simulink model "Bleed_TestBed1"  (R2019b)
settings: Solver=FixedStepDiscrete  StartTime=0.0  StopTime=1  FixedStep=1  RelTol=1e-3  EnableMultiTasking=on
undefined symbols (not defined in the file): MWS
libraries: Lib_Turbo_Bleed_TMATS x1
settings Model: Creator=jwchapm2  LastModifiedBy=bhisma
settings DataIOCC: LimitDataPoints=on  SaveFormat=Array  ReturnWorkspaceOutputs=off
settings OptimizationCC: ExpressionDepthLimit=2147483647  LifeSpan=inf
settings DebuggingCC: UnderspecifiedInitializationDetection=Classic  MergeDetectMultiDrivingBlocksExec=none  SolverPrmCheckMsg=warning  StateNameClashWarn=warning  SFUnexpectedBacktrackingDiag=warning  SFNoUnconditionalDefaultTransitionDiag=warning  SFExecutionAtInitializationDiag=none  ArithmeticOperatorsInVariantConditions=warning
settings HardwareCC: ProdBitPerPointer=32  ProdBitPerSizeT=32  ProdBitPerPtrDiffT=32  ProdLargestAtomicFloat=None  ProdIntDivRoundTo=Undefined  ProdEndianess=Unspecified  ProdWordSize=32  ProdHWDeviceType=32-bit Generic
settings ModelReferenceCC: PropagateSignalLabelsOutOfModel=off
settings SFSimCC: SimUseLocalCustomCode=off  CustomCodeUndefinedFunction=UseInterfaceOnly
settings RTWCC: RTWUseLocalCustomCode=off
settings CodeAppCC: StateflowObjectComments=on
settings GRTTargetCC: TargetLangStandard=C89/C90 (ANSI)  GeneratePreprocessorConditionals=Disable all
settings ConfigComp: CovMetricSettings=dw  CovHtmlReporting=on  CovSaveCumulativeToWorkspaceVar=on  CovSaveSingleToWorkspaceVar=on  CovExternalEMLEnable=off

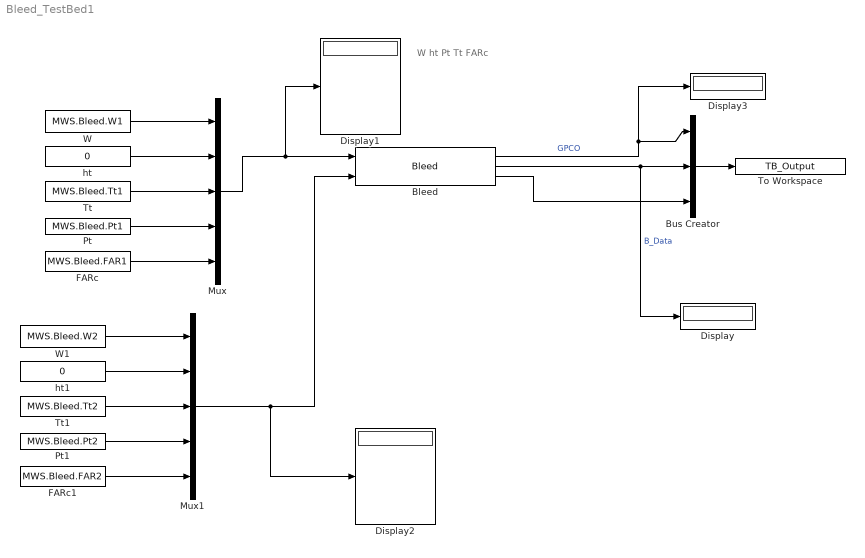
== system Bleed_TestBed1 ==
  note: W
      | ht
      | Pt
      | Tt
      | FARc
  Bleed : Lib_Turbo_Bleed_TMATS/Bleed  Wfrac_M=MWS.Bleed.W  BlkNm_M=0
  Bus Creator : BusCreator  Inputs=3
  Display{,1..3} (4 alike) : Display
  FARc : Constant  Value=MWS.Bleed.FAR1
  FARc1 : Constant  Value=MWS.Bleed.FAR2
  Mux : Mux  Inputs=5
  Mux1 : Mux  Inputs=5
  Pt : Constant  Value=MWS.Bleed.Pt1
  Pt1 : Constant  Value=MWS.Bleed.Pt2
  To Workspace : ToWorkspace  VariableName=TB_Output  SampleTime=-1
  Tt : Constant  Value=MWS.Bleed.Tt1
  Tt1 : Constant  Value=MWS.Bleed.Tt2
  W : Constant  Value=MWS.Bleed.W1
  W1 : Constant  Value=MWS.Bleed.W2
  ht : Constant  Value=0
  ht1 : Constant  Value=0
  wires:
  Bleed/1 -> Display3/1, Bus Creator/1  "GPCO"
  Bleed/2 -> Display/1, Bus Creator/2  "B_Data"
  Bus Creator/1 -> To Workspace/1
  W/1 -> Mux/1
  FARc/1 -> Mux/5
  Tt/1 -> Mux/3
  Pt/1 -> Mux/4
  Mux/1 -> Bleed/1, Display1/1
  ht/1 -> Mux/2
  Mux1/1 -> Display2/1, Bleed/2
  W1/1 -> Mux1/1
  FARc1/1 -> Mux1/5
  Tt1/1 -> Mux1/3
  Pt1/1 -> Mux1/4
  ht1/1 -> Mux1/2
  Bleed/3 -> Bus Creator/3
